simulink model "DGEN380_BO_2015a"  (R2015a)
settings: Solver=ode3  StartTime=0.0  StopTime=Tf  FixedStep=Te  RelTol=1e-3
values from neighbouring files (symbols this model uses):
  Cmd_kero_f = Cmd_kero_i+Cmd_kero_delta    (= 50)    [simulation_DGEN380.m]
  Cmd_kero_i = 50    [simulation_DGEN380.m]
  Cmd_kero_t = 200    [simulation_DGEN380.m]
  h = 2000    [simulation_DGEN380.m]
  T = 1    [simulation_DGEN380.m]
  v = 0.2    [simulation_DGEN380.m]
undefined symbols (not defined in the file or in its folder): SIMMOT_WESTT_CS
settings Model: CovSFcnEnable=off  Creator=Alexandre TAYMANS  LastModifiedBy=chfarges
settings DataIOCC: SignalLoggingSaveFormat=ModelDataLogs
settings OptimizationCC: ExpressionDepthLimit=2147483647
settings DebuggingCC: UnderspecifiedInitializationDetection=Classic  MergeDetectMultiDrivingBlocksExec=none  SolverPrmCheckMsg=warning  FcnCallInpInsideContextMsg=EnableAllAsWarning  StateNameClashWarn=warning
settings GRTTargetCC: TargetLangStandard=C99 (ISO)

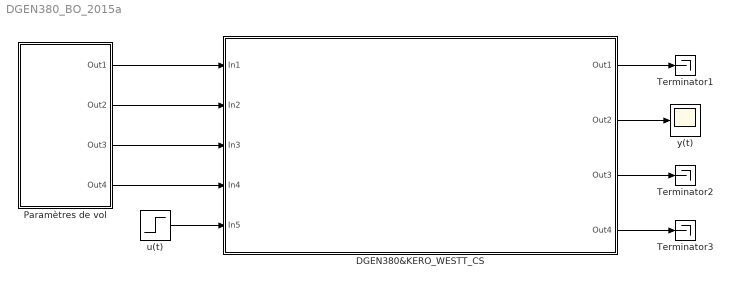
== system DGEN380_BO_2015a ==
  DGEN380&KERO_WESTT_CS : Subsystem  InitFcn=|
      | breakpointssave=dbstatus('SIMMOT_WESTT_CS');
      | clear SIMMOT_WESTT_CS;                      
      | dbstop(breakpointssave);                    
      | clear breakpointssave;
      mask help:
      | Unités des entrées:
      | Z = [m]
      | Mn = Mach Number
      | DTISA = [°C]
      | PWX = [W]
      | Cmd Kero = [%]
      | --------------------
      | Unités des sorties:
      | NH = [rpm]
      | NL = [rpm]
      | EGT = [K]
      | P3 = [Pa]
      mask Display:
      | image(imread('DGEN380.png'))
      | port_label('input',1,'z')
      | port_label('input',2,'mn')
      | port_label('input',3,'dtisa')
      | port_label('input',4,'pwx')
      | port_label('input',5,'cmd_kero')
      | 
      | port_label('output',1,'nh')
      | port_label('output',2,'nl')
      | port_label('output',3,'egt')
      | port_label('output',4,'p3')
  Paramètres de vol : Subsystem
      mask Display:
      | port_label('output',1,'Altitude')
      | port_label('output',2,'Vitesse')
      | port_label('output',3,'Température')
      | port_label('output',4,'Puiss.Elec.')
  Terminator1 : Terminator
  Terminator2 : Terminator
  Terminator3 : Terminator
  u(t) : Step  Time=Cmd_kero_t  Before=Cmd_kero_i  After=Cmd_kero_f
  y(t) : Scope
      settings: TimeRange=auto  MaxDataPoints=5000  SaveName=NL  YMin=37893.6  YMax=41882.4  SampleTime=-1
  wires:
  Paramètres de vol/1(Out1) -> DGEN380&KERO_WESTT_CS/1(In1)
  Paramètres de vol/2(Out2) -> DGEN380&KERO_WESTT_CS/2(In2)
  Paramètres de vol/3(Out3) -> DGEN380&KERO_WESTT_CS/3(In3)
  Paramètres de vol/4(Out4) -> DGEN380&KERO_WESTT_CS/4(In4)
  DGEN380&KERO_WESTT_CS/1(Out1) -> Terminator1/1
  u(t)/1 -> DGEN380&KERO_WESTT_CS/5(In5)
  DGEN380&KERO_WESTT_CS/2(Out2) -> y(t)/1
  DGEN380&KERO_WESTT_CS/3(Out3) -> Terminator2/1
  DGEN380&KERO_WESTT_CS/4(Out4) -> Terminator3/1

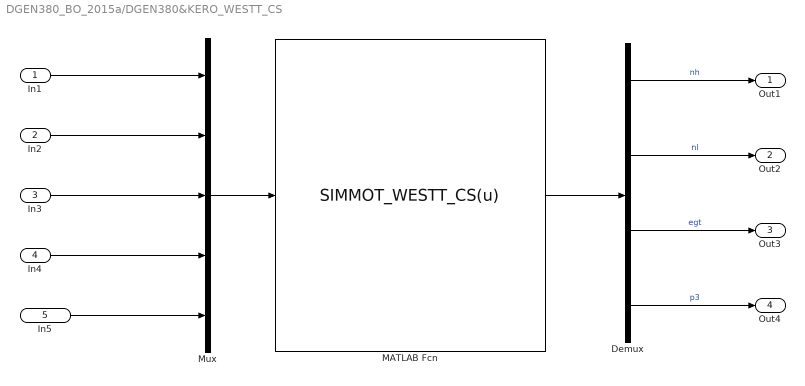
== system DGEN380_BO_2015a/DGEN380&KERO_WESTT_CS ==
  In1 : Inport
  In2 : Inport  Port=2
  In3 : Inport  Port=3
  In4 : Inport  Port=4
  In5 : Inport  Port=5
  Demux : Demux
  MATLAB Fcn : MATLABFcn  InitFcn=clear simmot  MATLABFcn=SIMMOT_WESTT_CS(u)  OutputDimensions=4
  Mux : Mux  Inputs=5
  Out1 : Outport
  Out2 : Outport  Port=2
  Out3 : Outport  Port=3
  Out4 : Outport  Port=4
  wires:
  Mux/1 -> MATLAB Fcn/1
  MATLAB Fcn/1 -> Demux/1
  Demux/1 -> Out1/1  "nh"
  Demux/2 -> Out2/1  "nl"
  Demux/3 -> Out3/1  "egt"
  Demux/4 -> Out4/1  "p3"
  In5/1 -> Mux/5
  In1/1 -> Mux/1
  In2/1 -> Mux/2
  In3/1 -> Mux/3
  In4/1 -> Mux/4

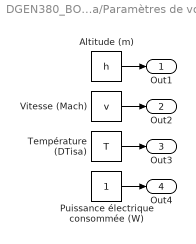
== system DGEN380_BO_2015a/Paramètres de vol ==
  Altitude (m) : Constant  Value=h
  Puissance électrique consommée (W) : Constant
  Température (DTisa) : Constant  Value=T
  Vitesse (Mach) : Constant  Value=v
  Out1 : Outport
  Out2 : Outport  Port=2
  Out3 : Outport  Port=3
  Out4 : Outport  Port=4
  wires:
  Altitude (m)/1 -> Out1/1
  Vitesse (Mach)/1 -> Out2/1
  Température (DTisa)/1 -> Out3/1
  Puissance électrique consommée (W)/1 -> Out4/1
